simulink model "Mohinhphanh1Acquy"  (R2024b)
settings: Solver=FixedStepAuto  StartTime=0  StopTime=2.08  FixedStep=0.0001  RelTol=1e-3  AbsTol=1e-3  EnableMultiTasking=on
values from neighbouring files (symbols this model uses):
  a01 = 0.2657    [Dulieuphanh.m]
  a02 = 0.0601    [Dulieuphanh.m]
  a11 = 0.060773449736866    (= 0.0607734497369)    [Dulieuphanh.m]
  a12 = 0.007150245075987    (= 0.00715024507599)    [Dulieuphanh.m]
  b01 = 6.7129    [Dulieuphanh.m]
  b02 = 8.2494    [Dulieuphanh.m]
  b11 = 1.576434187120628    (= 1.57643418712)    [Dulieuphanh.m]
  b12 = 0.153671177646358    (= 0.153671177646)    [Dulieuphanh.m]
  J_bx = 0.2412    [Dulieuphanh.m]
  J_cl = 1.2576    [Dulieuphanh.m]
  K = 1    [Dulieuphanh.m]
  r_bx = 0.245    [Dulieuphanh.m]
  r_cl = 0.1    [Dulieuphanh.m]
  Trr = 0.334273249247759    (= 0.334273249248)    [Dulieuphanh.m]
undefined symbols (not defined in the file or in its folder): h, km, m, rad, s
libraries: aerolibconvert2 x3, SignalEditorBlockLib x1
settings Model: Creator=Admin  LastModifiedBy=Legion
settings SolverCC: AutoScaleAbsTol=off  AlgebraicLoopSolver=TrustRegion  MaxZcPerStep=1
settings DataIOCC: LimitDataPoints=on  MaxDataPoints=10000
settings OptimizationCC: ReuseModelBlockBuffer=off  LifeSpan=inf
settings DebuggingCC: UnconnectedInputMsg=warning  UnconnectedOutputMsg=warning  UnconnectedLineMsg=warning  AllowSymbolicDim=off  SubsystemReferenceDiagnosticForUnitTest=warning  SFUnexpectedBacktrackingDiag=warning  SFNoUnconditionalDefaultTransitionDiag=warning  SFExecutionAtInitializationDiag=none  ArithmeticOperatorsInVariantConditions=warning
settings ModelReferenceCC: EnableRefExpFcnMdlSchedulingChecks=on
settings SFSimCC: SimUseLocalCustomCode=off  CustomCodeUndefinedFunction=UseInterfaceOnly
settings RTWCC: RTWUseLocalCustomCode=off  GPUComputeCapability=3.5  DLArmComputeVersion=19.05
settings CodeAppCC: StateflowObjectComments=on
settings GRTTargetCC: TargetLangStandard=C89/C90 (ANSI)
settings ConfigComp: CovMetricSettings=dw  CovSaveCumulativeToWorkspaceVar=on  CovSaveSingleToWorkspaceVar=on  CovExternalEMLEnable=off  CovSFcnEnable=off
settings SimscapeCC: SimscapeLogType=all  SimscapeLogSimulationStatistics=on  SimscapeLogDataHistory=10000

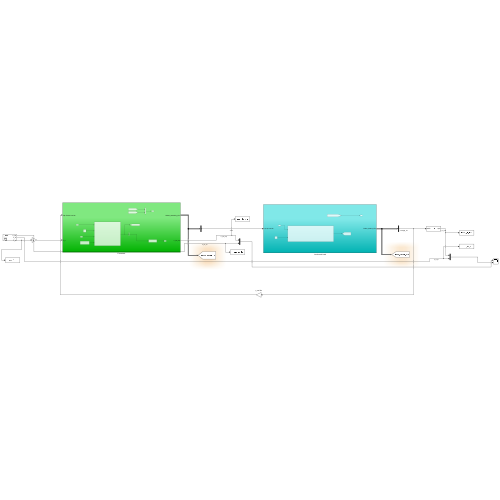
[thumbnail: Simulink's stored preview of the top-level diagram]
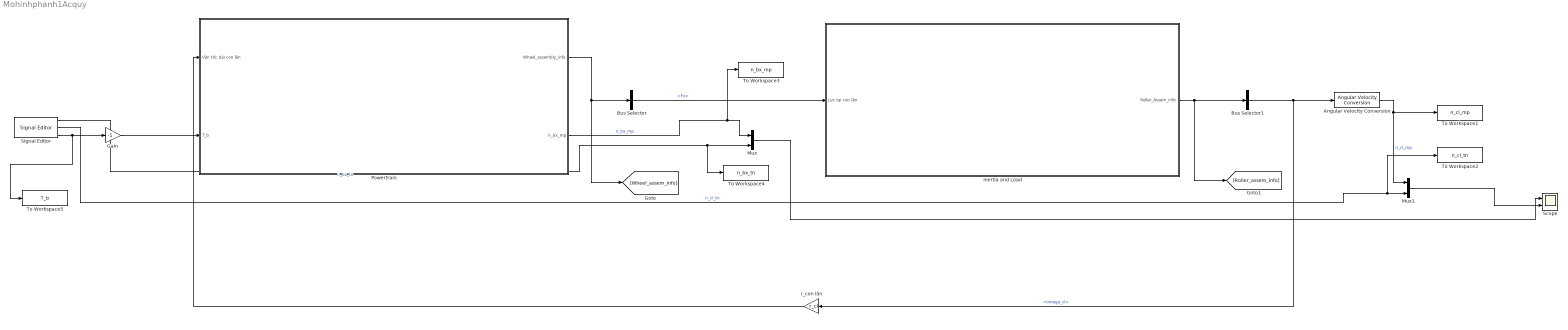
== system Mohinhphanh1Acquy ==
  " Inertia and Load" : Subsystem
  Angular Velocity Conversion : aerolibconvert2/Angular Velocity Conversion  IU=rad/s  OU=rpm
  Bus Selector : BusSelector  OutputSignals=Wheel info.Fx
  Bus Selector1 : BusSelector  OutputSignals=omega_cl
  Gain : Gain  Gain=-1
  Mux : Mux  Inputs=2
  Mux1 : Mux  Inputs=2
  Powertrain : Subsystem
  Scope : Scope  NumInputPorts=2
  Signal Editor : SignalEditorBlockLib/Signal Editor  FileName=DataPhanh1acquy.mat  ActiveScenario=Sheet1  ActiveSignal=n_bx  IsBus=off  OutputBusObjectStr=Bus: BusObject  SampleTime=0  ZeroCross=off  OutputAfterFinalValue=Setting to zero  Unit=inherit  PreserveSignalName=on  ApplySigPropsToAllScenarios=on  ApplySigPropsToAllSignals=off
  To Workspace1 : ToWorkspace  VariableName=n_cl_mp  SaveFormat=Timeseries  SampleTime=-1
  To Workspace2 : ToWorkspace  VariableName=n_cl_tn  SaveFormat=Timeseries  SampleTime=-1
  To Workspace3 : ToWorkspace  VariableName=n_bx_mp  SaveFormat=Timeseries  SampleTime=-1
  To Workspace4 : ToWorkspace  VariableName=n_bx_tn  SaveFormat=Timeseries  SampleTime=-1
  To Workspace5 : ToWorkspace  VariableName=T_b  SaveFormat=Timeseries  SampleTime=-1
  r_con lăn : Gain  Gain=r_cl
  wires:
  Bus Selector/1 -> " Inertia and Load"/1(Lực tại con lăn)  "<Fx>"
  Powertrain/1(Wheel_assembly_info) -> Bus Selector/1, [Wheel_assem_info]
  " Inertia and Load"/1(Roller_Assem_info) -> [Roller_assem_info], Bus Selector1/1
  Bus Selector1/1 -> r_con lăn/1, Angular Velocity Conversion/1  "<omega_cl>"
  r_con lăn/1 -> Powertrain/1(Vận tốc dài con lăn)
  Powertrain/2(n_bx_mp) -> To Workspace3/1, Mux/1  "n_bx_mp"
  Angular Velocity Conversion/1 -> Mux1/1, To Workspace1/1  "n_cl_mp"
  Mux/1 -> Scope/1
  Signal Editor/3 -> To Workspace5/1, Gain/1
  Gain/1 -> Powertrain/2(T_b)
  Signal Editor/2 -> To Workspace2/1, Mux1/2  "n_cl_tn"
  Signal Editor/1 -> To Workspace4/1, Mux/2  "n_bx_tn"
  Mux1/1 -> Scope/2

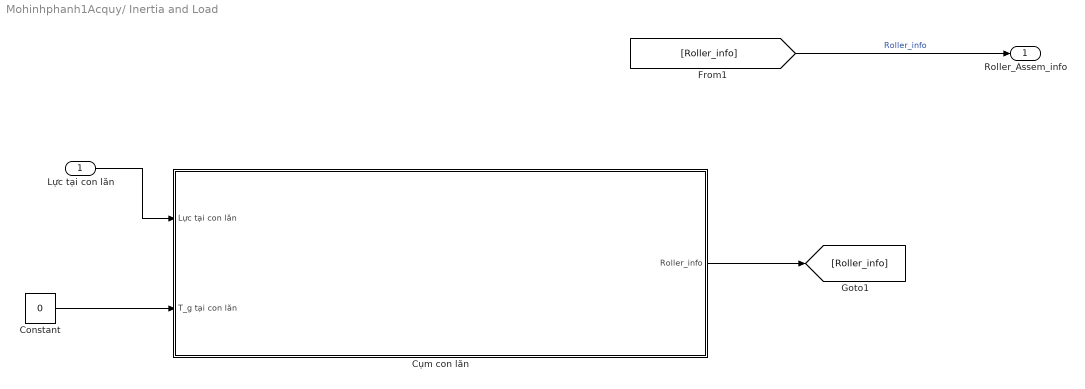
== system Mohinhphanh1Acquy/ Inertia and Load ==
  Lực tại con lăn : Inport
  Constant : Constant  Value=0
  Cụm con lăn : Subsystem
  Roller_Assem_info : Outport
  wires:
  Lực tại con lăn/1 -> Cụm con lăn/1(Lực tại con lăn)
  Cụm con lăn/1(Roller_info) -> [Roller_info]
  [Roller_info] -> Roller_Assem_info/1  "Roller_info"
  Constant/1 -> Cụm con lăn/2(T_g tại con lăn)

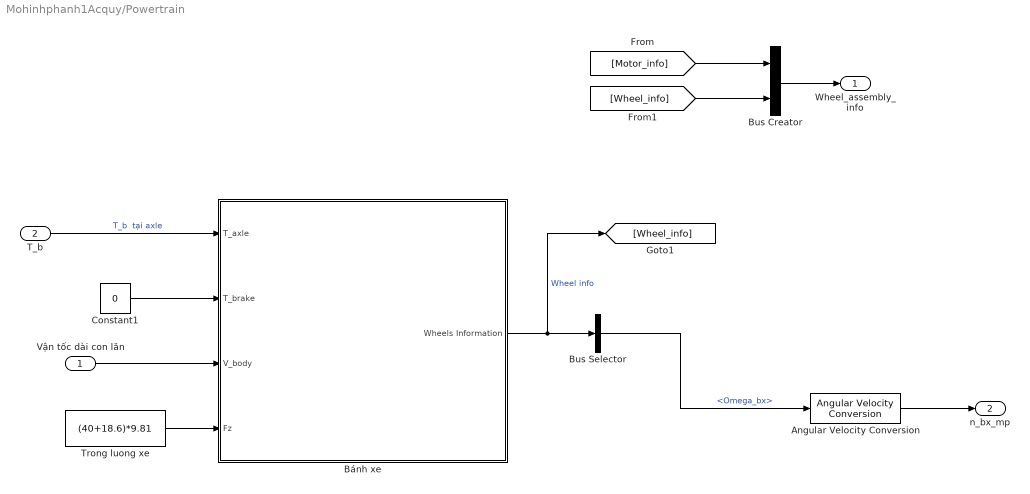
== system Mohinhphanh1Acquy/Powertrain ==
  Vận tốc dài con lăn : Inport
  T_b : Inport  Port=2
  Angular Velocity Conversion : aerolibconvert2/Angular Velocity Conversion  IU=rad/s  OU=rpm
  Bus Creator : BusCreator  Inputs=2
  Bus Selector : BusSelector  OutputSignals=Omega_bx
  Bánh xe : Subsystem
  Constant1 : Constant  Value=0
  Trong luong xe : Constant  Value=(40+18.6)*9.81
  Wheel_assembly_info : Outport
  n_bx_mp : Outport  Port=2
  wires:
  Bánh xe/1(Wheels Information) -> [Wheel_info], Bus Selector/1  "Wheel info"
  T_b/1 -> Bánh xe/1(T_axle)  "T_b  tại axle"
  Trong luong xe/1 -> Bánh xe/4(Fz)
  Constant1/1 -> Bánh xe/2(T_brake)
  Bus Selector/1 -> Angular Velocity Conversion/1  "<Omega_bx>"
  Vận tốc dài con lăn/1 -> Bánh xe/3(V_body)
  [Motor_info] -> Bus Creator/1
  [Wheel_info] -> Bus Creator/2
  Bus Creator/1 -> Wheel_assembly_info/1
  Angular Velocity Conversion/1 -> n_bx_mp/1

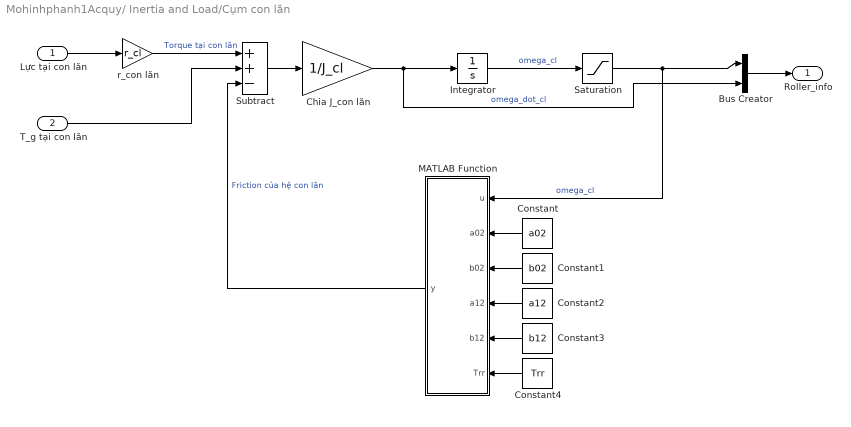
== system Mohinhphanh1Acquy/ Inertia and Load/Cụm con lăn ==
  Lực tại con lăn : Inport
  T_g tại con lăn : Inport  Port=2
  Bus Creator : BusCreator  Inputs=2
  Chia J_con lăn : Gain  Gain=1/J_cl
  Constant : Constant  Value=a02
  Constant1 : Constant  Value=b02
  Constant2 : Constant  Value=a12
  Constant3 : Constant  Value=b12
  Constant4 : Constant  Value=Trr
  Integrator : Integrator  InitialCondition=39.4364
  MATLAB Function : MATLAB Function  TreatAsAtomicUnit=on
  Saturation : Saturate  UpperLimit=inf  LowerLimit=0
  Subtract : Sum  Inputs=++-
  r_con lăn : Gain  Gain=r_cl
  Roller_info : Outport
  wires:
  Subtract/1 -> Chia J_con lăn/1
  r_con lăn/1 -> Subtract/1  "Torque tại con lăn"
  Saturation/1 -> Bus Creator/1, MATLAB Function/1(u)  "omega_cl"
  Integrator/1 -> Saturation/1  "omega_cl"
  Chia J_con lăn/1 -> Bus Creator/2, Integrator/1  "omega_dot_cl"
  MATLAB Function/1(y) -> Subtract/3  "Friction của hệ con lăn"
  T_g tại con lăn/1 -> Subtract/2
  Lực tại con lăn/1 -> r_con lăn/1
  Bus Creator/1 -> Roller_info/1
  Constant/1 -> MATLAB Function/2(a02)
  Constant1/1 -> MATLAB Function/3(b02)
  Constant2/1 -> MATLAB Function/4(a12)
  Constant3/1 -> MATLAB Function/5(b12)
  Constant4/1 -> MATLAB Function/6(Trr)

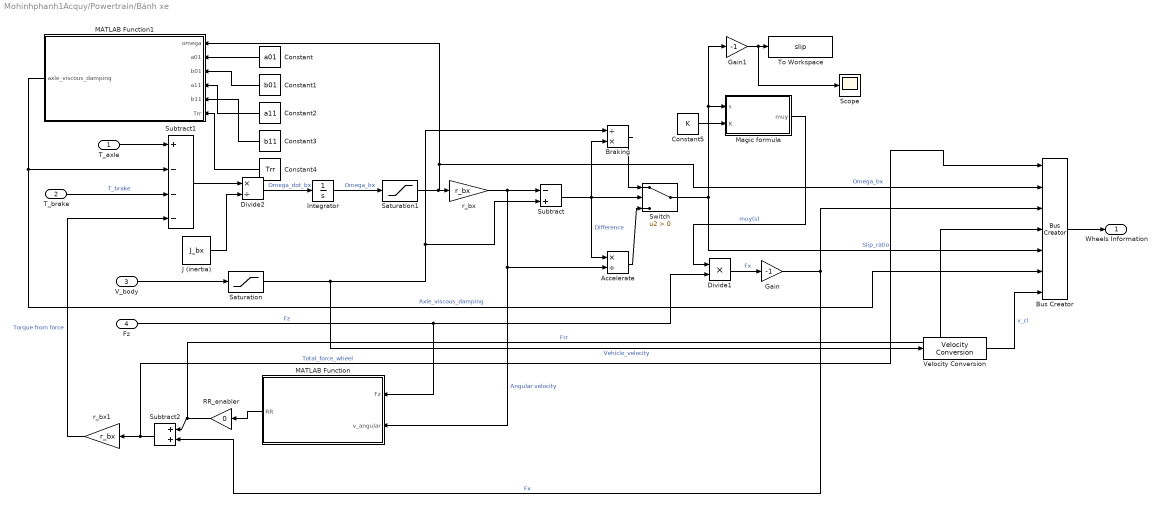
== system Mohinhphanh1Acquy/Powertrain/Bánh xe ==
  T_axle : Inport
  T_brake : Inport  Port=2
  V_body : Inport  Port=3
  Fz : Inport  Port=4
  Accelerate : Product  Inputs=*/
  Braking : Product  Inputs=/*
  Bus Creator : BusCreator  Inputs=7
  Constant : Constant  Value=a01
  Constant1 : Constant  Value=b01
  Constant2 : Constant  Value=a11
  Constant3 : Constant  Value=b11
  Constant4 : Constant  Value=Trr
  Constant5 : Constant  Value=K
  Divide1 : Product  Inputs=**
  Divide2 : Product  Inputs=*/
  Gain : Gain  Gain=-1
  Gain1 : Gain  Gain=-1
  Integrator : Integrator  InitialCondition=16.3518
  J (inertia) : Constant  Value=J_bx
  MATLAB Function : MATLAB Function  TreatAsAtomicUnit=on
  MATLAB Function1 : MATLAB Function  TreatAsAtomicUnit=on
  Magic formula : MATLAB Function  TreatAsAtomicUnit=on
  RR_enabler : Gain  Gain=0
  Saturation : Saturate  UpperLimit=inf  LowerLimit=0.00000000000000001
  Saturation1 : Saturate  UpperLimit=inf  LowerLimit=0.00000000000000001  ZeroCross=off
  Scope : Scope
  Subtract : Sum  Inputs=-+
  Subtract1 : Sum  Inputs=+---
  Subtract2 : Sum
  Switch : Switch  Criteria=u2 > Threshold  SaturateOnIntegerOverflow=off  InputSameDT=off
  To Workspace : ToWorkspace  VariableName=slip  SaveFormat=Timeseries  SampleTime=-1
  Velocity Conversion : aerolibconvert2/Velocity Conversion  IU=m/s  OU=km/h
  r_bx : Gain  Gain=r_bx
  r_bx1 : Gain  Gain=r_bx
  Wheels Information : Outport
  wires:
  Fz/1 -> Divide1/2, MATLAB Function/1(Fz)  "Fz"
  Subtract/1 -> Switch/2, Accelerate/1, Braking/2  "Difference"
  Saturation/1 -> Velocity Conversion/1, Braking/1, Subtract/2  "Vehicle_velocity"
  T_axle/1 -> Subtract1/1
  T_brake/1 -> Subtract1/3  "T_brake"
  Magic formula/1(muy) -> Divide1/1  "muy(s)"
  Accelerate/1 -> Switch/3
  Braking/1 -> Switch/1
  Switch/1 -> Bus Creator/5, Gain1/1, Magic formula/1(s)  "Slip_ratio"
  Subtract1/1 -> Divide2/1
  J (inertia)/1 -> Divide2/2
  Divide2/1 -> Integrator/1  "Omega_dot_bx"
  Divide1/1 -> Gain/1  "Fx"
  Gain/1 -> Bus Creator/3, Subtract2/2  "Fx"
  V_body/1 -> Saturation/1
  r_bx/1 -> Subtract/1, Accelerate/2, MATLAB Function/2(v_angular)  "Angular velocity"
  RR_enabler/1 -> Bus Creator/4, Subtract2/1  "Frr"
  MATLAB Function/1(RR) -> RR_enabler/1
  Subtract2/1 -> Bus Creator/1, r_bx1/1  "Total_force_wheel"
  r_bx1/1 -> Subtract1/4  "Torque from force"
  Saturation1/1 -> Bus Creator/2, MATLAB Function1/1(omega), r_bx/1  "Omega_bx"
  MATLAB Function1/1(axle_viscous_damping) -> Subtract1/2, Bus Creator/6  "Axle_viscous_damping"
  Integrator/1 -> Saturation1/1  "Omega_bx"
  Bus Creator/1 -> Wheels Information/1
  Velocity Conversion/1 -> Bus Creator/7  "v_cl"
  Constant/1 -> MATLAB Function1/2(a01)
  Constant1/1 -> MATLAB Function1/3(b01)
  Constant2/1 -> MATLAB Function1/4(a11)
  Constant3/1 -> MATLAB Function1/5(b11)
  Constant4/1 -> MATLAB Function1/6(Trr)
  Constant5/1 -> Magic formula/2(K)
  Gain1/1 -> Scope/1, To Workspace/1

== matlab function Mohinhphanh1Acquy/Powertrain/Bánh xe/MATLAB Function ==
  data: Fz input; RR output; v_angular input
function RR = rolling_resistance_function(Fz,v_angular)

RR = (0.015+7*10^(-6)*v_angular^2)*Fz;

== matlab function Mohinhphanh1Acquy/Powertrain/Bánh xe/Magic formula ==
  data: s input; muy output; K input
function muy = magicformula(s, K)
% Khai báo hằng số mặt đường
B = 12;
C = 2.3;
D = 0.82;
E = 1;
% Magic formula
muy = K * D * sin(C * atan(B * s - E * (B * s - atan(B * s))));

== matlab function Mohinhphanh1Acquy/Powertrain/Bánh xe/MATLAB Function1 ==
  data: omega input; axle_viscous_damping output; a01 input; b01 input; a11 input; b11 input; Trr input
function axle_viscous_damping = fcn(omega, a01, b01, a11, b11, Trr)
    axle_viscous_damping=0.0362*(a01*(omega)+b01)*15 + (a11*omega + b11) + Trr;

== matlab function Mohinhphanh1Acquy/ Inertia and Load/Cụm con lăn/MATLAB Function ==
  data: u input; y output; a02 input; b02 input; a12 input; b12 input; Trr input
function y = fcn(u,a02,b02,a12,b12,Trr)

y = 0.0362*(a02*u+b02)*2 + (a12*u+b12) + Trr;
